simulink model "Speed Controlled Two Quadrant DC Motor Drive"  (R2023b)
settings: Solver=VariableStepAuto  StartTime=0.0  StopTime=10.0  RelTol=1e-3
undefined symbols (not defined in the file): Bt, Hc, J, Kb, Kc, Ks, Kw, La, Ra, Tc, Ts, Tw
libraries: simulink_extras x6, spsVoltageMeasurementLib x4, spsACVoltageSourceLib x3, spsUniversalBridgeLib x1, spsGroundLib x1, spsParallelRLCBranchLib x1, sps_lib x1
settings Model: Creator=USER  LastModifiedBy=USER

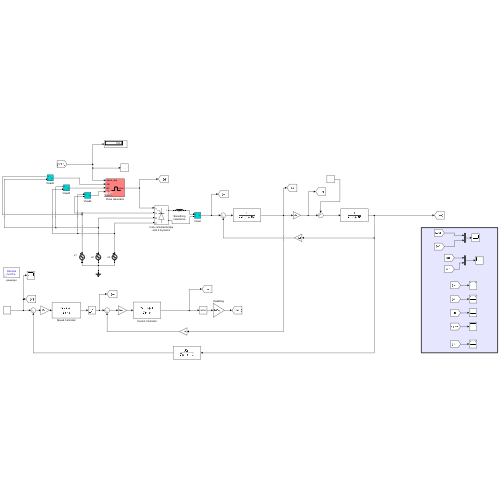
[thumbnail: Simulink's stored preview of the top-level diagram]
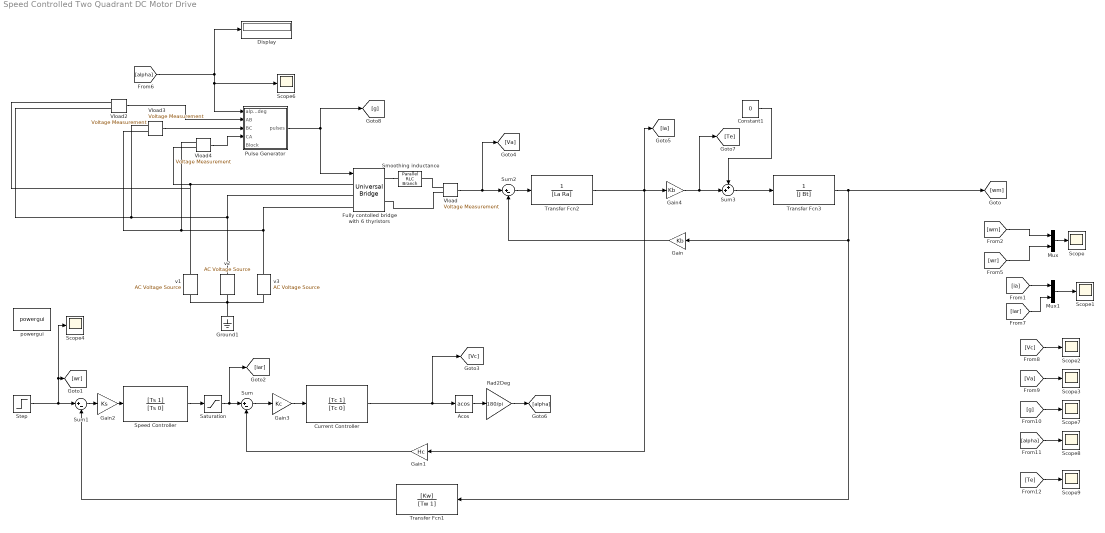
== system Speed Controlled Two Quadrant DC Motor Drive ==
  Acos : Trigonometry  Operator=acos
  Constant1 : Constant  Value=0
  Current Controller : TransferFcn  Numerator=[Tc 1]  Denominator=[Tc 0]
  Display : Display
  Fully contolled bridge with 6 thyristors : spsUniversalBridgeLib/Universal Bridge  Arms=3  SnubberResistance=1e5  SnubberCapacitance=inf  Device=Thyristors  Ron=1e-3  Lon=0  ForwardVoltages="[  0  0  ]"  ForwardVoltage=0  GTOparameters=[ 10e-6 , 20e-6 ]  IGBTparameters=[ 1e-6 , 2e-6 ]  Measurements=None  Measurements_2=None  converterType=Rectifier
  Gain : Gain  Gain=Kb
  Gain1 : Gain  Gain=Hc
  Gain2 : Gain  Gain=Ks
  Gain3 : Gain  Gain=Kc
  Gain4 : Gain  Gain=Kb
  Ground1 : spsGroundLib/Ground  LConnTagsString=a
  Mux : Mux  Inputs=2
  Mux1 : Mux  Inputs=2
  Pulse Generator : Subsystem  AncestorBlock=|  DialogController=POWERSYS.PowerSysDialog  mask(Synchronized 6-pulse generator){freq=60, pwidth=60, Double_Pulse=off}
      | powerlib_extras/Control 
      | Blocks/Synchronized
      | 6-Pulse Generator
      mask prompts: freq "Frequency of synchronisation voltages (Hz) :"; pwidth "Pulse width (degrees) :"; Double_Pulse "Double pulsing"
      mask help: Use this block to fire the 6 thyristors of a 6-pulse converter. The output is a vector of 6 pulses (0-1) individually synchronized on the 6 commutation voltages. Pulses are generated alpha degrees after the increasing zero-crossings of the commutation voltages.
      mask init:
      | power_initmask();
      mask Help: helpview(psbhelp)
      mask Display: plot(0,0,100,100,[80 62 62 47 47 30],[40 40 60 60 40 40]-5)
  Rad2Deg : Gain  Gain=180/pi  SaturateOnIntegerOverflow=on  OutDataTypeStr=Inherit: Same as input  ParamDataTypeStr=Inherit: Same as input
  Saturation : Saturate  UpperLimit=10  LowerLimit=0
  Scope{,1..4,6..9} (9 alike) : Scope
  Smoothing inductance : spsParallelRLCBranchLib/Parallel RLC Branch  LConnTagsString=a  RConnTagsString=__new0  BranchType=L  Resistance=[]  Inductance=15e-3  SetiL0=off  InitialCurrent=0  Capacitance=[]  Setx0=off  InitialVoltage=0  Measurements=None
  Speed Controller : TransferFcn  Numerator=[Ts 1]  Denominator=[Ts 0]
  Step : Step  SampleTime=0
  Sum : Sum  Inputs=|+-
  Sum1 : Sum  Inputs=|+-
  Sum2 : Sum  Inputs=|+-
  Sum3 : Sum  Inputs=++|
  Transfer Fcn1 : TransferFcn  Numerator=[Kw]  Denominator=[Tw 1]
  Transfer Fcn2 : TransferFcn  Denominator=[La Ra]
  Transfer Fcn3 : TransferFcn  Denominator=[J Bt]
  Vload{,2..4} (4 alike) : spsVoltageMeasurementLib/Voltage Measurement  PhasorSimulation=off  OutputType=Complex  PSBequivalent=0
  powergui : sps_lib/powergui  Priority=1  SimulationMode=Discrete  SampleTime=50e-6  frequency=60  Iterations=50  frequencyindice=0  Pbase=100e6  ErrMax=1e-4  UnitsV=kV  UnitsW=MW  buscounter=0  FunctionMessages=off  echomessages=off  EnableUseOfTLC=off  CurrentSourceSwitches=off  DisableSnubberDevices=off  DisableRonSwitches=off  DisableVfSwitches=off  DisplayEquations=off  AutomaticDiscreteSolvers=off  SolverType=Tustin/Backward Euler (TBE)  Interpol=off  ExternalGateDelay=off  methode=off  Ts=10  x0status=blocks  SPID=off  SwTol=0  HookPort=off  NonlinearTolerance=1e-4  nMaxIteration=100  ContinueOnMaxIteration=off  RestoreLinks=warning  ResistiveCurrentMeasurement=off  Frange=[0:2:500]  Ylog=off  Xlog=on  ShowGrid=off  save=off  variable=ZData  structure=0  ZoomFFT=off  StartTime=0.0  cycles=1  DisplayStyle=1  fundamental=60  FreqAxis=off  MaxFrequency=1000  frequencyindicesteady=1  RmsSteady=1  display=off
  "v1 " : spsACVoltageSourceLib/AC Voltage Source  Amplitude=220  Phase=0  Frequency=60  SampleTime=0  Measurements=Voltage  BusType=swing  Pref=10e3  Qref=0  Qmin=-inf  Qmax=+inf
  v2 : spsACVoltageSourceLib/AC Voltage Source  Amplitude=220  Phase=-120  Frequency=60  SampleTime=0  Measurements=Voltage  BusType=swing  Pref=10e3  Qref=0  Qmin=-inf  Qmax=+inf
  v3 : spsACVoltageSourceLib/AC Voltage Source  Amplitude=220  Phase=120  Frequency=60  SampleTime=0  Measurements=Voltage  BusType=swing  Pref=10e3  Qref=0  Qmin=-inf  Qmax=+inf
  wires:
  Sum/1 -> Gain3/1
  Transfer Fcn1/1 -> Sum1/2
  Step/1 -> Scope4/1, [wr], Sum1/1
  Gain3/1 -> Current Controller/1
  Saturation/1 -> [iar], Sum/1
  Speed Controller/1 -> Saturation/1
  Sum1/1 -> Gain2/1
  Transfer Fcn3/1 -> Transfer Fcn1/1, Gain/1, [wm]
  Gain1/1 -> Sum/2
  Gain2/1 -> Speed Controller/1
  Pulse Generator/1(pulses) -> Fully contolled bridge with 6 thyristors/1, [g]
  Vload4/1 -> Pulse Generator/4(CA)
  Vload3/1 -> Pulse Generator/3(BC)
  [alpha] -> Pulse Generator/1(alpha_deg), Scope6/1, Display/1
  Vload2/1 -> Pulse Generator/2(AB)
  Sum2/1 -> Transfer Fcn2/1
  Gain/1 -> Sum2/2
  Gain4/1 -> [Te], Sum3/2
  Constant1/1 -> Sum3/1
  Transfer Fcn2/1 -> Gain1/1, [ia], Gain4/1
  Vload/1 -> [Va], Sum2/1
  Acos/1 -> Rad2Deg/1
  Rad2Deg/1 -> [alpha]
  Sum3/1 -> Transfer Fcn3/1
  Current Controller/1 -> [Vc], Acos/1
  [wr] -> Mux/2
  [Te] -> Scope9/1
  [iar] -> Mux1/2
  Mux1/1 -> Scope1/1
  [Vc] -> Scope2/1
  Mux/1 -> Scope/1
  [g] -> Scope7/1
  [wm] -> Mux/1
  [ia] -> Mux1/1
  [alpha] -> Scope8/1
  [Va] -> Scope3/1
  connections:
  Vload3/LConn2 -- v3/RConn1 -- Fully contolled bridge with 6 thyristors/LConn3 -- Vload4/LConn1
  v2/LConn1 -- v3/LConn1 -- Ground1/LConn1 -- "v1 "/LConn1
  Vload2/LConn2 -- v2/RConn1 -- Fully contolled bridge with 6 thyristors/LConn2 -- Vload3/LConn1
  Vload4/LConn2 -- Fully contolled bridge with 6 thyristors/LConn1 -- "v1 "/RConn1 -- Vload2/LConn1
  Vload/LConn2 -- Fully contolled bridge with 6 thyristors/RConn2
  Fully contolled bridge with 6 thyristors/RConn1 -- Smoothing inductance/LConn1
  Vload/LConn1 -- Smoothing inductance/RConn1

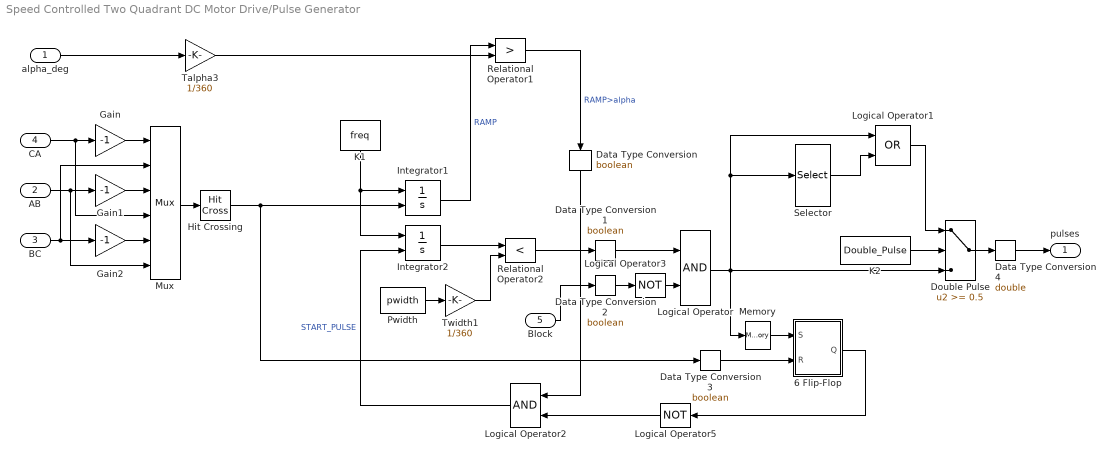
== system Speed Controlled Two Quadrant DC Motor Drive/Pulse Generator ==
  alpha_deg : Inport
  AB : Inport  Port=2
  BC : Inport  Port=3
  CA : Inport  Port=4
  Block : Inport  Port=5
  6 Flip-Flop : Subsystem
  Data Type Conversion{,1..3} (4 alike) : DataTypeConversion  OutDataTypeStr=boolean
  Data Type Conversion4 : DataTypeConversion  OutDataTypeStr=double
  Double Pulse : Switch  Threshold=0.5  SaturateOnIntegerOverflow=off
  Gain : Gain  Gain=-1  SaturateOnIntegerOverflow=on  OutDataTypeStr=Inherit: Same as input  ParamDataTypeStr=Inherit: Same as input
  Gain1 : Gain  Gain=-1  SaturateOnIntegerOverflow=on  OutDataTypeStr=Inherit: Same as input  ParamDataTypeStr=Inherit: Same as input
  Gain2 : Gain  Gain=-1  SaturateOnIntegerOverflow=on  OutDataTypeStr=Inherit: Same as input  ParamDataTypeStr=Inherit: Same as input
  Hit Crossing : HitCross  HitCrossingDirection=rising
  Integrator1 : Integrator  ExternalReset=rising
  Integrator2 : Integrator  ExternalReset=rising
  K1 : Constant  Value=freq
  K2 : Constant  Value=Double_Pulse
  Logical Operator : Logic
  Logical Operator1 : Logic  Operator=OR
  Logical Operator2 : Logic
  Logical Operator3 : Logic  Operator=NOT  Inputs=1
  Logical Operator5 : Logic  Operator=NOT  Inputs=1
  Memory : Memory
  Mux : Mux  Inputs=6
  Pwidth : Constant  Value=pwidth
  Relational Operator1 : RelationalOperator  Operator=>
  Relational Operator2 : RelationalOperator  Operator=<
  Selector : Selector  InputPortWidth=6  IndexOptions=Index vector (dialog)  Indices=[2 3 4 5 6 1 ]  OutputSizes=1
  Talpha3 : Gain  Gain=1/360  SaturateOnIntegerOverflow=on  OutDataTypeStr=Inherit: Same as input  ParamDataTypeStr=Inherit: Same as input
  Twidth1 : Gain  Gain=1/360  SaturateOnIntegerOverflow=on  OutDataTypeStr=Inherit: Same as input  ParamDataTypeStr=Inherit: Same as input
  pulses : Outport  InitialOutput=0
  wires:
  Data Type Conversion4/1 -> pulses/1
  Double Pulse/1 -> Data Type Conversion4/1
  Logical Operator1/1 -> Double Pulse/1
  Data Type Conversion3/1 -> 6 Flip-Flop/2(R)
  Data Type Conversion2/1 -> Logical Operator3/1
  Block/1 -> Data Type Conversion2/1
  Data Type Conversion1/1 -> Logical Operator/1
  Relational Operator2/1 -> Data Type Conversion1/1
  Data Type Conversion/1 -> Logical Operator2/1
  Relational Operator1/1 -> Data Type Conversion/1  "RAMP>alpha"
  Selector/1 -> Logical Operator1/2
  Logical Operator/1 -> Double Pulse/3, Logical Operator1/1, Selector/1, Memory/1
  K2/1 -> Double Pulse/2
  Memory/1 -> 6 Flip-Flop/1(S)
  Integrator1/1 -> Relational Operator1/1  "RAMP"
  Talpha3/1 -> Relational Operator1/2
  Integrator2/1 -> Relational Operator2/1
  Twidth1/1 -> Relational Operator2/2
  Logical Operator3/1 -> Logical Operator/2
  6 Flip-Flop/1(Q) -> Logical Operator5/1
  Logical Operator2/1 -> Integrator2/2  "START_PULSE"
  Logical Operator5/1 -> Logical Operator2/2
  Hit Crossing/1 -> Data Type Conversion3/1, Integrator1/2
  Pwidth/1 -> Twidth1/1
  K1/1 -> Integrator2/1, Integrator1/1
  Mux/1 -> Hit Crossing/1
  AB/1 -> Mux/6, Gain1/1
  CA/1 -> Mux/4, Gain/1
  BC/1 -> Mux/2, Gain2/1
  Gain2/1 -> Mux/5
  Gain1/1 -> Mux/3
  Gain/1 -> Mux/1
  alpha_deg/1 -> Talpha3/1

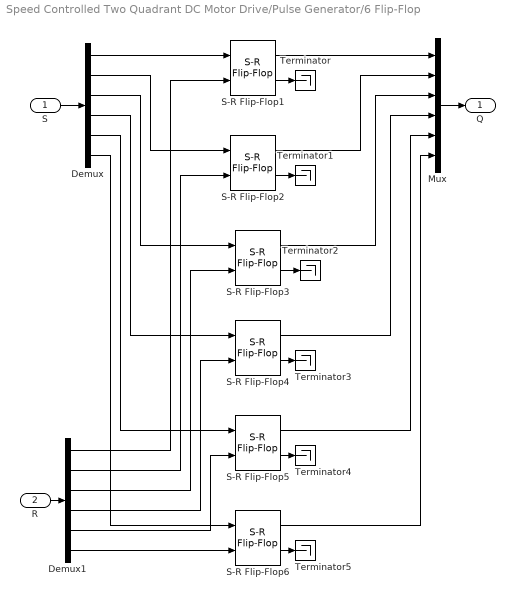
== system Speed Controlled Two Quadrant DC Motor Drive/Pulse Generator/6 Flip-Flop ==
  S : Inport
  R : Inport  Port=2
  Demux : Demux  Outputs=6
      settings: DisplayOption=none
  Demux1 : Demux  Outputs=6
      settings: DisplayOption=none
  Mux : Mux  Inputs=6
  S-R Flip-Flop{1..6} (6 alike) : simulink_extras/Flip Flops/S-R Flip-Flop  initial_condition=0
  Terminator{,1..5} (6 alike) : Terminator
  Q : Outport
  wires:
  Demux1/6 -> S-R Flip-Flop6/2
  Demux1/5 -> S-R Flip-Flop5/2
  Demux1/4 -> S-R Flip-Flop4/2
  Demux1/3 -> S-R Flip-Flop3/2
  Demux1/2 -> S-R Flip-Flop2/2
  Demux1/1 -> S-R Flip-Flop1/2
  R/1 -> Demux1/1
  Demux/5 -> S-R Flip-Flop5/1
  Demux/6 -> S-R Flip-Flop6/1
  S/1 -> Demux/1
  Demux/4 -> S-R Flip-Flop4/1
  Demux/3 -> S-R Flip-Flop3/1
  Demux/2 -> S-R Flip-Flop2/1
  Demux/1 -> S-R Flip-Flop1/1
  S-R Flip-Flop1/2 -> Terminator/1
  S-R Flip-Flop6/1 -> Mux/6
  Mux/1 -> Q/1
  S-R Flip-Flop5/1 -> Mux/5
  S-R Flip-Flop4/1 -> Mux/4
  S-R Flip-Flop3/1 -> Mux/3
  S-R Flip-Flop2/1 -> Mux/2
  S-R Flip-Flop1/1 -> Mux/1
  S-R Flip-Flop2/2 -> Terminator1/1
  S-R Flip-Flop3/2 -> Terminator2/1
  S-R Flip-Flop4/2 -> Terminator3/1
  S-R Flip-Flop5/2 -> Terminator4/1
  S-R Flip-Flop6/2 -> Terminator5/1
